simulink model "px4_6dof_quadrotor"  (R2021b)
settings: Solver=VariableStepAuto  StartTime=0.0  StopTime=10.0  RelTol=1e-3
undefined symbols (not defined in the file or in its folder): DiscIntNeverNeededParam, magnitude, rad, s
libraries: cstblocks x6, aerolibconvert2 x4, simulink x3, simulink_extras x3, sharedtransform x1, mspfiltlib x1, mspsensorlib x1
settings Model: Creator=user  LastModifiedBy=user

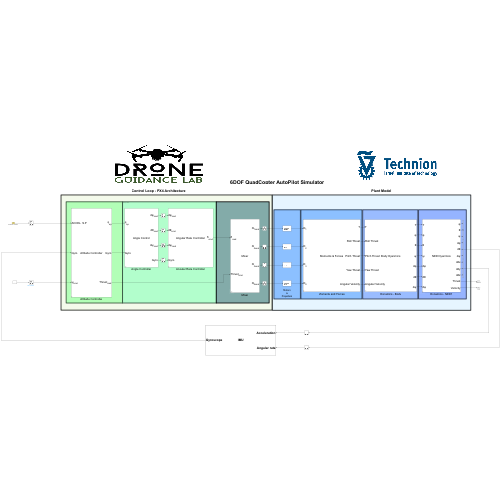
[thumbnail: Simulink's stored preview of the top-level diagram]
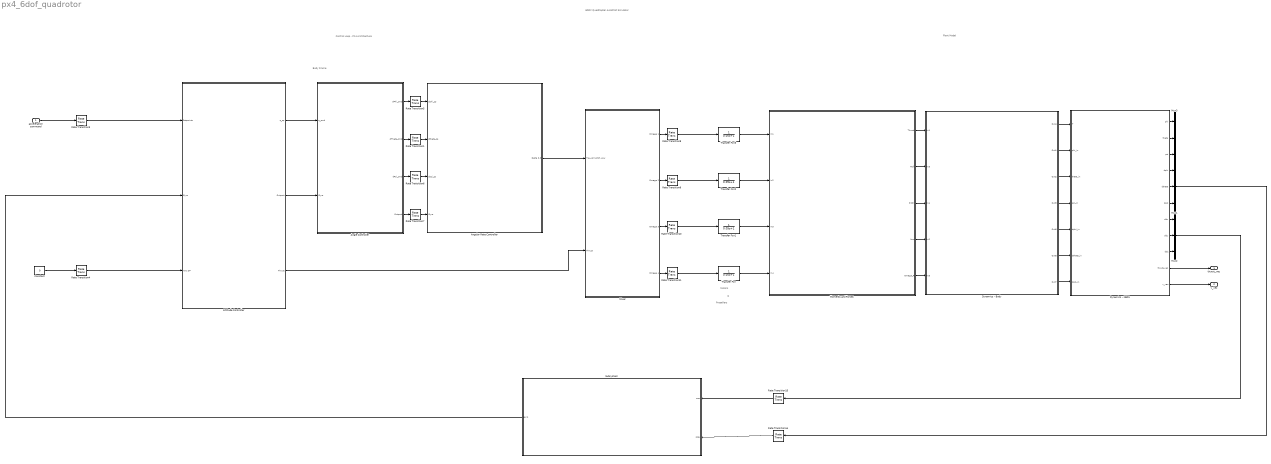
== system px4_6dof_quadrotor ==
  note: Control Loop - PX4 Architecture
  note: Body Frame
  note: Motors
  note: Plant Model
  note: 6DOF QuadCopter AutoPilot Simulator
  note: &
  note: Propellers
  acceleration command : Inport
  Angle Controller : Subsystem  mask{MC_ROLL_P=4, MC_PITCH_P=4, MC_YAW_P=4, MC_ROLLRATE_MAX=2, MC_PITCHRATE_MAX=2, MC_YAWRATE_MAX=2, MC_ACRO_R_MAX=2, MC_YAW_WEIGHT=0.1, m=0.9}
      mask prompts: MC_ROLL_P "MC_ROLL_P ="; MC_PITCH_P "MC_PITCH_P ="; MC_YAW_P "MC_YAW_P ="; MC_ROLLRATE_MAX "MC_ROLLRATE_MAX ="; MC_PITCHRATE_MAX "MC_PITCHRATE_MAX ="; MC_YAWRATE_MAX "MC_YAWRATE_MAX ="; MC_ACRO_R_MAX "MC_ACRO_R_MAX ="; MC_YAW_WEIGHT "MC_YAW_WEIGHT ="; m "m [kg] ="
      mask DialogControl DescTextVar Prompt: Attitude Controller - based on PX4 architecture
      mask Display:
      | disp('Angle Control')
      | 
      | port_label('input',1,'q_{sp}','texmode','on')
      | port_label('input',2,'Gyro')
      | 
      | port_label('output',1,'d\phi_{cmd}','texmode','on')
      | port_label('output',2,'d\theta_{cmd}','texmode','on')
      | port_label('output',3,'d\psi_{cmd}','texmode','on')
      | port_label('output',4,'Gyro','texmode','on')
  Angular Rate Controller : Subsystem  mask{MC_ROLLRATE_K=1, MC_ROLLRATE_P=0.044, MC_ROLLRATE_I=0.05, MC_ROLLRATE_D=0.0012, MC_RR_INT_LIM=101, MC_PITCHRATE_K=1, MC_PITCHRATE_P=0.044, MC_PITCHRATE_I=0.05, MC_PITCHRATE_D=0.0012, MC_PR_INT_LIM=100, MC_YAWRATE_K=1, MC_YAWRATE_P=0.044, MC_YAWRATE_I=0.05, MC_YAWRATE_D=0.0012, MC_YR_INT_LIM=100, IMU_DGYRO_CUTOFF=6000, IMU_GYRO_CUTOFF=0}
      mask prompts: MC_ROLLRATE_K "MC_ROLLRATE_K ="; MC_ROLLRATE_P "MC_ROLLRATE_P ="; MC_ROLLRATE_I "MC_ROLLRATE_I ="; MC_ROLLRATE_D "MC_ROLLRATE_D ="; MC_RR_INT_LIM "MC_RR_INT_LIM ="; MC_PITCHRATE_K "MC_PITCHRATE_K ="; MC_PITCHRATE_P "MC_PITCHRATE_P ="; MC_PITCHRATE_I "MC_PITCHRATE_I ="; MC_PITCHRATE_D "MC_PITCHRATE_D ="; MC_PR_INT_LIM "MC_PR_INT_LIM ="; MC_YAWRATE_K "MC_YAWRATE_K ="; MC_YAWRATE_P "MC_YAWRATE_P ="; MC_YAWRATE_I "MC_YAWRATE_I ="; MC_YAWRATE_D "MC_YAWRATE_D ="; MC_YR_INT_LIM "MC_YR_INT_LIM ="; IMU_DGYRO_CUTOFF "IMU_DGYRO_CUTOFF ="; IMU_GYRO_CUTOFF "IMU_GYRO_CUTOFF ="
      mask DialogControl DescTextVar Prompt: Angular rate controller, based on PX4 architecture
      mask DialogControl ROLL Prompt: Roll
      mask DialogControl PITCH Prompt: Pitch
      mask DialogControl YAW Prompt: Yaw
      mask Display:
      | disp('Angular Rate Controller')
      | 
      | port_label('input',1,'d\phi_{cmd}','texmode','on')
      | port_label('input',2,'d\theta_{cmd}','texmode','on')
      | port_label('input',3,'d\psi_{cmd}','texmode','on')
      | port_label('input',4,'Gyro','texmode','on')
      | 
      | port_label('output',1,'\delta_{cmd}','texmode','on')
  Attitude Controller : Subsystem  mask{MC_ROLL_P=1, MC_PITCH_P=5, MC_YAW_P=1, MC_ROLLRATE_MAX=2, MC_PITCHRATE_MAX=2, MC_YAWRATE_MAX=2, MC_ACRO_R_MAX=2, MC_YAW_WEIGHT=0.1, m=0.9}
      mask prompts: MC_ROLL_P "MC_ROLL_P ="; MC_PITCH_P "MC_PITCH_P ="; MC_YAW_P "MC_YAW_P ="; MC_ROLLRATE_MAX "MC_ROLLRATE_MAX ="; MC_PITCHRATE_MAX "MC_PITCHRATE_MAX ="; MC_YAWRATE_MAX "MC_YAWRATE_MAX ="; MC_ACRO_R_MAX "MC_ACRO_R_MAX ="; MC_YAW_WEIGHT "MC_YAW_WEIGHT ="; m "m [kg] ="
      mask DialogControl DescTextVar Prompt: Attitude Controller - based on PX4 architecture
      mask Display:
      | disp('Attitude Controller')
      | 
      | port_label('input',1,'ACCEL. S.P')
      | port_label('input',2,'Gyro')
      | port_label('input',3,'\psi_{cmd}','texmode','on')
      | 
      | port_label('output',1,'q_{sp}','texmode','on')
      | port_label('output',2,'Gyro','texmode','on')
      | port_label('output',3,'Thrust_{cmd}','texmode','on')
  Constant : Constant  Value=0
  Dynamics - Body : Subsystem  mask{Ixx=0.001, Iyy=0.001, Izz=0.0015, Jr=8e-7, d=0.165}
      mask prompts: Ixx "Ixx [kg*m^2] ="; Iyy "Iyy [kg*m^2] ="; Izz "Izz [kg*m^2]="; Jr "Jl [kg*m^2]="; d "d [m] ="
      mask DialogControl DescTextVar Prompt: This model represents the body-frame dyanmics. Enter the MOIs of the system
      mask Display:
      | disp('Body Dyanmics','texmode','on')
      | 
      | port_label('input',1,'T','texmode','on')
      | port_label('input',2,'Roll Thrust','texmode','on')
      | port_label('input',3,'Pitch Thrust','texmode','on')
      | port_label('input',4,'Yaw Thrust','texmode','on')
      | port_label('input',5,'Angular Velocity','texmode','on')
      | 
      | port_label('output',2,'\phi','texmode','on')
      | port_label('output',3,'\theta','texmode','on')
      | port_label('output',4,'\psi','texmode','on')
      | port_label('output',1,'T','texmode','on')
      | port_label('output',5,'d\phi','texmode','on')
      | port_label('output',6,'d\theta','texmode','on')
      | port_label('output',7,'d\psi','texmode','on')
  Dynamics - NED1 : Subsystem  mask{g=9.81, m=0.9, k=0.9}
      mask prompts: g "g [m/s^2] ="; m "m [kg] ="; k "k ="
      mask DialogControl DescTextVar Prompt: This block transform the body dyanmics to NED. Choose the mass, gravity, and Ax,Ay,Az - drag coeff.
      mask Display:
      | disp('NED Dyanmics','texmode','on')
      | 
      | port_label('input',2,'\phi','texmode','on')
      | port_label('input',3,'\theta','texmode','on')
      | port_label('input',4,'\psi','texmode','on')
      | port_label('input',1,'T','texmode','on')
      | port_label('input',5,'d\phi','texmode','on')
      | port_label('input',6,'d\theta','texmode','on')
      | port_label('input',7,'d\psi','texmode','on')
      | 
      | % port_label('output',1,'X','texmode','on')
      | % port_label('output',2,'Y','texmode','on')
      | % port_label('output',3,'Z','texmode','on')
      | 
      | % port_label('output',4,'dX','texmode','on')
      | % port_label('output',5,'dY','texmode','on')
      | % port_label('output',6,'dZ','texmode','on')
      | 
      | port_label('output',7,'ddx','texmode','on')
      | port_label('output',8,'ddy','texmode','on')
      | port_label('output',9,'ddz','texmode','on')
      | 
      | port_label('output',4,'d\phi','texmode','on')
      | port_label('output',5,'d\theta','texmode','on')
      | port_label('output',6,'d\psi','texmode','on')
      | 
      | port_label('output',1,'\phi','texmode','on')
      | port_label('output',2,'\theta','texmode','on')
      | port_label('output',3,'\psi','texmode','on')
      | 
      | port_label('output',10,'Thrust','texmode','on')
      | port_label('output',11,'Velocity','texmode','on')
  Mixer : Subsystem  mask{Ct=7e-6, Cq=1.6e-7, d=0.165}
      mask prompts: Ct "Ct ="; Cq "Cq ="; d "d [m] ="
      mask Display:
      | disp('Mixer')
      | 
      | port_label('input',1,'\delta_{cmd}','texmode','on')
      | port_label('input',2,'Thrust_{cmd}','texmode','on')
      | 
      | port_label('output',1,'\Omega_{1cmd}','texmode','on')
      | port_label('output',2,'\Omega_{2cmd}','texmode','on')
      | port_label('output',3,'\Omega_{3cmd}','texmode','on')
      | port_label('output',4,'\Omega_{4cmd}','texmode','on')
  Moments and Forces : Subsystem  mask{Ct=7e-6, Cq=1.6e-7, d=0.165, rpm_sat=15000}
      mask prompts: Ct "Ct ="; Cq "Cq ="; d "d [m] ="; rpm_sat "max motor speed [rpm]="
      mask DialogControl DescTextVar Prompt: This block represents the moment and force calculations. Supply the Ct - thrust constant and Cq is the drag consant. d is the quadrotor arm's length
      mask DialogControl Container3 Prompt: Constants:
      mask Display:
      | disp('Moments & Forces')
      | 
      | port_label('input',1,'\Omega_{1}','texmode','on')
      | port_label('input',2,'\Omega_{2}','texmode','on')
      | port_label('input',3,'\Omega_{3}','texmode','on')
      | port_label('input',4,'\Omega_{4}','texmode','on')
      | 
      | port_label('output',1,'T','texmode','on')
      | port_label('output',2,'Roll Thrust','texmode','on')
      | port_label('output',3,'Pitch Thrust','texmode','on')
      | port_label('output',4,'Yaw Thrust','texmode','on')
      | port_label('output',5,'Angular Velocity','texmode','on')
  Mux1 : Mux  Inputs=3
  Mux2 : Mux  Inputs=3
  Mux3 : Mux  Inputs=3
  Rate Transition{1,5..7} (4 alike) : RateTransition  OutPortSampleTime=1/1000
  Rate Transition{8..11} (4 alike) : RateTransition  OutPortSampleTime=1/10000
  Rate Transition14 : RateTransition  OutPortSampleTime=1/250
  Rate Transition15 : RateTransition  OutPortSampleTime=1/250
  Rate Transition3 : RateTransition  OutPortSampleTime=1/250
  Rate Transition4 : RateTransition  OutPortSampleTime=1/ 250
  Subsystem : Subsystem
      mask Display:
      | disp('IMU')
      | port_label('input',1,'Acceleration','texmode','on')
      | port_label('input',2,'Angular rate','texmode','on')
      | port_label('output',1,'Gyroscope','texmode','on')
  Transfer Fcn{,1..3} (4 alike) : TransferFcn  Denominator=[0.05 1]
  thurst_vec : Outport
  v_vec : Outport  Port=2
  wires:
  Moments and Forces/1(Thrust) -> Dynamics - Body/1(In1)
  Transfer Fcn/1 -> Moments and Forces/4(In4)
  Rate Transition15/1 -> Subsystem/1(acc)
  Mux1/1 -> Rate Transition14/1
  Subsystem/1(gyro) -> Attitude Controller/2(Gyro)
  Dynamics - NED1/1(phi) -> Mux3/1
  Dynamics - NED1/6(dpsi) -> Mux1/3
  Attitude Controller/2(Outport) -> Angle Controller/2(Gyro)
  Rate Transition9/1 -> Transfer Fcn2/1
  Dynamics - NED1/2(theta) -> Mux3/2
  Mixer/1(Omega 1) -> Rate Transition8/1
  Rate Transition10/1 -> Transfer Fcn1/1
  Dynamics - NED1/4(dphi) -> Mux1/1
  Dynamics - NED1/9(ddz) -> Mux2/3
  Rate Transition14/1 -> Subsystem/2(rate)
  Rate Transition5/1 -> Angular Rate Controller/1(dphi_sp)
  Angle Controller/2(dTheta_cmd) -> Rate Transition1/1
  Rate Transition6/1 -> Angular Rate Controller/3(dpsi_sp)
  Dynamics - NED1/5(dtheta) -> Mux1/2
  Angle Controller/3(dPsi_cmd) -> Rate Transition6/1
  Rate Transition3/1 -> Attitude Controller/1(Setpoints)
  Dynamics - NED1/3(psi) -> Mux3/3
  Transfer Fcn1/1 -> Moments and Forces/3(In3)
  Rate Transition11/1 -> Transfer Fcn/1
  Transfer Fcn3/1 -> Moments and Forces/1(In1)
  Transfer Fcn2/1 -> Moments and Forces/2(In2)
  Dynamics - Body/4(Out3) -> Dynamics - NED1/4(psi_in)
  Moments and Forces/5(Omega_R) -> Dynamics - Body/5(In5)
  Rate Transition1/1 -> Angular Rate Controller/2(dtheta_sp)
  Mixer/3(Omega 3) -> Rate Transition10/1
  Rate Transition4/1 -> Attitude Controller/3(Yaw.SP)
  acceleration command/1 -> Rate Transition3/1
  Dynamics - Body/1(Out4) -> Dynamics - NED1/1(T)
  Dynamics - NED1/8(ddy) -> Mux2/2
  Attitude Controller/1(q_sp) -> Angle Controller/1(q_cmd)
  Constant/1 -> Rate Transition4/1
  Dynamics - Body/7(Out7) -> Dynamics - NED1/7(dpsi_in)
  Angular Rate Controller/1(Delta S.P) -> Mixer/1(Tau_roll,pitch,yaw)
  Moments and Forces/4(Yaw) -> Dynamics - Body/4(In2)
  Angle Controller/4(Outport) -> Rate Transition7/1
  Dynamics - Body/6(Out6) -> Dynamics - NED1/6(dtheta_in)
  Rate Transition8/1 -> Transfer Fcn3/1
  Dynamics - Body/5(Out5) -> Dynamics - NED1/5(dphi_in)
  Mixer/4(Omega 4) -> Rate Transition11/1
  Dynamics - NED1/11(v_vec) -> v_vec/1
  Dynamics - NED1/10(thrust_vec) -> thurst_vec/1
  Attitude Controller/3(Thrust) -> Mixer/2(Thrust)
  Dynamics - NED1/7(ddx) -> Mux2/1
  Moments and Forces/3(Pitch) -> Dynamics - Body/3(In4)
  Dynamics - Body/3(Out2) -> Dynamics - NED1/3(theta_in)
  Mixer/2(Omega 2) -> Rate Transition9/1
  Moments and Forces/2(Roll) -> Dynamics - Body/2(In3)
  Mux2/1 -> Rate Transition15/1
  Angle Controller/1(dPhi_cmd) -> Rate Transition5/1
  Dynamics - Body/2(Out1) -> Dynamics - NED1/2(phi_in)
  Rate Transition7/1 -> Angular Rate Controller/4(Gyro)

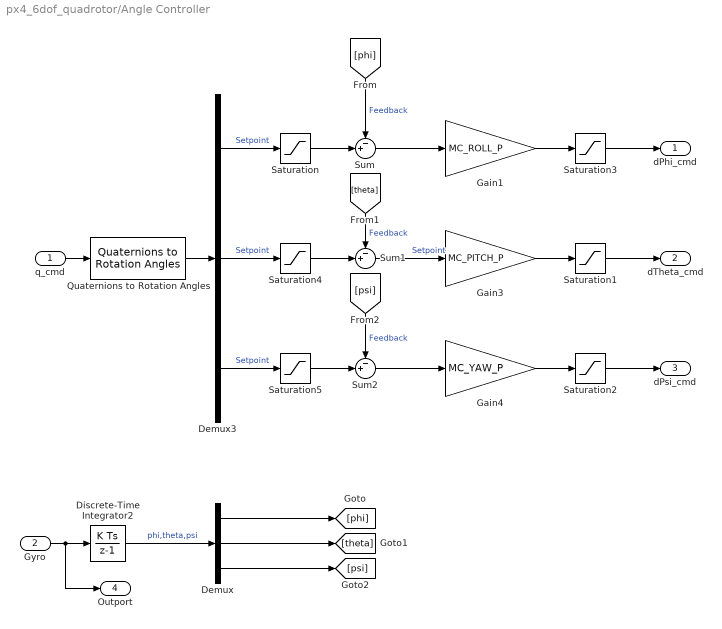
== system px4_6dof_quadrotor/Angle Controller ==
  q_cmd : Inport
  Gyro : Inport  Port=2
  Demux : Demux  Outputs=3
  Demux3 : Demux  Outputs=3
  Discrete-Time Integrator2 : DiscreteIntegrator  InitialCondition=[0.001;0.001;0.001]  SampleTime=-1  ICPrevOutput=DiscIntNeverNeededParam  ICPrevScaledInput=DiscIntNeverNeededParam
  Gain1 : Gain  Gain=MC_ROLL_P
  Gain3 : Gain  Gain=MC_PITCH_P
  Gain4 : Gain  Gain=MC_YAW_P
  Quaternions to Rotation Angles : sharedtransform/Quaternions to Rotation Angles  rotationOrder=XYZ  aMode=aMode
      settings: SourceProductBaseCode=AE,PW,DR,MT,UV,VE
  Saturation : Saturate  UpperLimit=1.5  LowerLimit=-1.5
  Saturation1 : Saturate  UpperLimit=MC_PITCHRATE_MAX  LowerLimit=-MC_PITCHRATE_MAX
  Saturation2 : Saturate  UpperLimit=MC_YAWRATE_MAX  LowerLimit=-MC_YAWRATE_MAX
  Saturation3 : Saturate  UpperLimit=MC_ROLLRATE_MAX  LowerLimit=-MC_ROLLRATE_MAX
  Saturation4 : Saturate  UpperLimit=1.5  LowerLimit=-1.5
  Saturation5 : Saturate  UpperLimit=1.5  LowerLimit=-1.5
  Sum : Sum  Inputs=-+|
  Sum1 : Sum  Inputs=-+|
  Sum2 : Sum  Inputs=-+|
  dPhi_cmd : Outport
  dTheta_cmd : Outport  Port=2
  dPsi_cmd : Outport  Port=3
  Outport : Outport  Port=4
  wires:
  Discrete-Time Integrator2/1 -> Demux/1  "phi,theta,psi"
  Gyro/1 -> Outport/1, Discrete-Time Integrator2/1
  Demux/2 -> [theta]
  Demux/1 -> [phi]
  Demux/3 -> [psi]
  Demux3/1 -> Saturation/1  "Setpoint"
  Demux3/2 -> Saturation4/1  "Setpoint"
  Demux3/3 -> Saturation5/1  "Setpoint"
  Saturation3/1 -> dPhi_cmd/1
  Gain1/1 -> Saturation3/1
  Gain3/1 -> Saturation1/1
  Gain4/1 -> Saturation2/1
  Saturation1/1 -> dTheta_cmd/1
  Saturation2/1 -> dPsi_cmd/1
  [phi] -> Sum/1  "Feedback"
  Sum/1 -> Gain1/1
  [theta] -> Sum1/1  "Feedback"
  Sum2/1 -> Gain4/1
  [psi] -> Sum2/1  "Feedback"
  Sum1/1 -> Gain3/1  "Setpoint"
  q_cmd/1 -> Quaternions to Rotation Angles/1
  Quaternions to Rotation Angles/1 -> Demux3/1
  Saturation/1 -> Sum/2
  Saturation4/1 -> Sum1/2
  Saturation5/1 -> Sum2/2

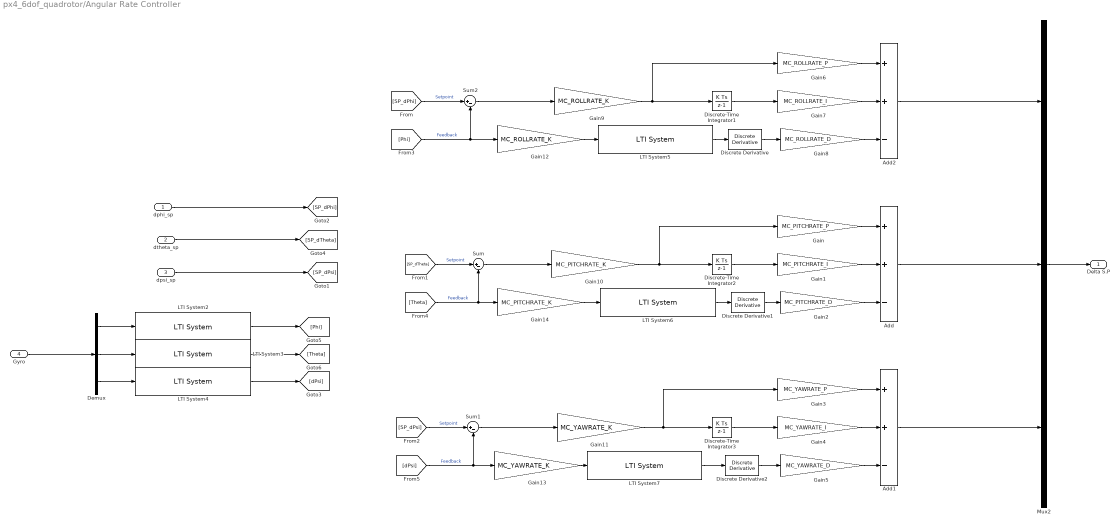
== system px4_6dof_quadrotor/Angular Rate Controller ==
  dphi_sp : Inport
  dtheta_sp : Inport  Port=2
  dpsi_sp : Inport  Port=3
  Gyro : Inport  Port=4
  Add : Sum  Inputs=++-
  Add1 : Sum  Inputs=++-
  Add2 : Sum  Inputs=++-
  Demux : Demux  Outputs=3
  Discrete Derivative : simulink/Discrete/Discrete Derivative  gainval=1.0  ICPrevScaledInput=0.0  OutMin=[]  OutMax=[]  OutDataType=fixdt(1, 16)  OutScaling=2^-10  DoSatur=off
  Discrete Derivative1 : simulink/Discrete/Discrete Derivative  gainval=1.0  ICPrevScaledInput=0.0  OutMin=[]  OutMax=[]  OutDataType=fixdt(1, 16)  OutScaling=2^-10  DoSatur=off
  Discrete Derivative2 : simulink/Discrete/Discrete Derivative  gainval=1.0  ICPrevScaledInput=0.0  OutMin=[]  OutMax=[]  OutDataType=fixdt(1, 16)  OutScaling=2^-10  DoSatur=off
  Discrete-Time Integrator1 : DiscreteIntegrator  SampleTime=1/1000  LimitOutput=on  UpperSaturationLimit=MC_RR_INT_LIM  LowerSaturationLimit=-MC_RR_INT_LIM  ICPrevOutput=DiscIntNeverNeededParam  ICPrevScaledInput=DiscIntNeverNeededParam
  Discrete-Time Integrator2 : DiscreteIntegrator  SampleTime=1/1000  LimitOutput=on  UpperSaturationLimit=MC_PR_INT_LIM  LowerSaturationLimit=-MC_PR_INT_LIM  ICPrevOutput=DiscIntNeverNeededParam  ICPrevScaledInput=DiscIntNeverNeededParam
  Discrete-Time Integrator3 : DiscreteIntegrator  SampleTime=1/1000  LimitOutput=on  UpperSaturationLimit=MC_YR_INT_LIM  LowerSaturationLimit=-MC_YR_INT_LIM  ICPrevOutput=DiscIntNeverNeededParam  ICPrevScaledInput=DiscIntNeverNeededParam
  Gain : Gain  Gain=MC_PITCHRATE_P
  Gain1 : Gain  Gain=MC_PITCHRATE_I
  Gain10 : Gain  Gain=MC_PITCHRATE_K
  Gain11 : Gain  Gain=MC_YAWRATE_K
  Gain12 : Gain  Gain=MC_ROLLRATE_K
  Gain13 : Gain  Gain=MC_YAWRATE_K
  Gain14 : Gain  Gain=MC_PITCHRATE_K
  Gain2 : Gain  Gain=MC_PITCHRATE_D
  Gain3 : Gain  Gain=MC_YAWRATE_P
  Gain4 : Gain  Gain=MC_YAWRATE_I
  Gain5 : Gain  Gain=MC_YAWRATE_D
  Gain6 : Gain  Gain=MC_ROLLRATE_P
  Gain7 : Gain  Gain=MC_ROLLRATE_I
  Gain8 : Gain  Gain=MC_ROLLRATE_D
  Gain9 : Gain  Gain=MC_ROLLRATE_K
  LTI System2 : cstblocks/LTI System  sys=c2d(tf(1,[IMU_GYRO_CUTOFF 1]),1/1000)  IC=[]
  LTI System3 : cstblocks/LTI System  sys=c2d(tf(1,[IMU_GYRO_CUTOFF 1]),1/1000)  IC=[]
  LTI System4 : cstblocks/LTI System  sys=c2d(tf(1,[IMU_GYRO_CUTOFF 1]),1/1000)  IC=[]
  LTI System5 : cstblocks/LTI System  sys=c2d(tf(1,[IMU_DGYRO_CUTOFF 1]),1/1000)  IC=[]
  LTI System6 : cstblocks/LTI System  sys=c2d(tf(1,[IMU_DGYRO_CUTOFF 1]),1/1000)  IC=[]
  LTI System7 : cstblocks/LTI System  sys=c2d(tf(1,[IMU_DGYRO_CUTOFF 1]),1/1000)  IC=[]
  Mux2 : Mux  Inputs=3
  Sum : Sum  Inputs=|+-
  Sum1 : Sum  Inputs=|+-
  Sum2 : Sum  Inputs=|+-
  Delta S.P : Outport
  wires:
  dtheta_sp/1 -> [SP_dTheta]
  LTI System6/1 -> Discrete Derivative1/1
  Sum/1 -> Gain10/1
  Discrete-Time Integrator2/1 -> Gain1/1
  Gain2/1 -> Add/3
  Gain1/1 -> Add/2
  Gain/1 -> Add/1
  Gain3/1 -> Add1/1
  Gain4/1 -> Add1/2
  Gain5/1 -> Add1/3
  Discrete-Time Integrator3/1 -> Gain4/1
  Sum1/1 -> Gain11/1
  LTI System7/1 -> Discrete Derivative2/1
  [dPsi] -> Gain13/1, Sum1/2  "Feedback"
  [SP_dPsi] -> Sum1/1  "Setpoint"
  Add/1 -> Mux2/2
  Mux2/1 -> Delta S.P/1
  Gain6/1 -> Add2/1
  Gain7/1 -> Add2/2
  Gain8/1 -> Add2/3
  Discrete-Time Integrator1/1 -> Gain7/1
  Sum2/1 -> Gain9/1
  LTI System5/1 -> Discrete Derivative/1
  [SP_dPhi] -> Sum2/1  "Setpoint"
  [SP_dTheta] -> Sum/1  "Setpoint"
  [Phi] -> Gain12/1, Sum2/2  "Feedback"
  [Theta] -> Gain14/1, Sum/2  "Feedback"
  Add1/1 -> Mux2/3
  Discrete Derivative/1 -> Gain8/1
  Discrete Derivative1/1 -> Gain2/1
  Discrete Derivative2/1 -> Gain5/1
  Gain9/1 -> Discrete-Time Integrator1/1, Gain6/1
  Gain10/1 -> Discrete-Time Integrator2/1, Gain/1
  Gain11/1 -> Discrete-Time Integrator3/1, Gain3/1
  Gain12/1 -> LTI System5/1
  Gain13/1 -> LTI System7/1
  Gain14/1 -> LTI System6/1
  Gyro/1 -> Demux/1
  Demux/1 -> LTI System2/1
  Demux/2 -> LTI System3/1
  Demux/3 -> LTI System4/1
  LTI System2/1 -> [Phi]
  LTI System3/1 -> [Theta]
  LTI System4/1 -> [dPsi]
  dpsi_sp/1 -> [SP_dPsi]
  dphi_sp/1 -> [SP_dPhi]
  Add2/1 -> Mux2/1

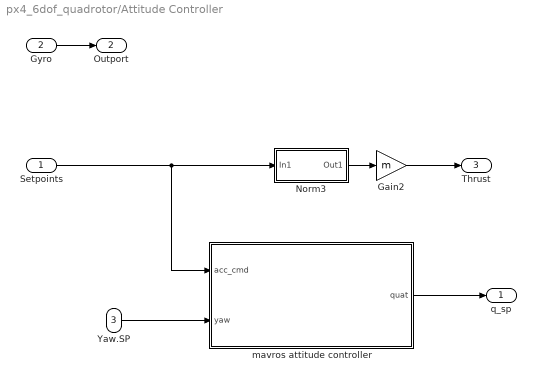
== system px4_6dof_quadrotor/Attitude Controller ==
  Setpoints : Inport
  Gyro : Inport  Port=2
  Yaw.SP : Inport  Port=3
  Gain2 : Gain  Gain=m
  Norm3 : Subsystem
      mask Display: disp('Norm')
  mavros attitude controller : Subsystem
      mask Display:
      | disp('Mavros Geometric controller')
      | port_label('input',1,'acc_{cmd}','texmode','on')
      | port_label('input',2,'\psi_{cmd}','texmode','on')
      | 
      | 
      | port_label('output',1,'quat','texmode','on')
  q_sp : Outport
  Outport : Outport  Port=2
  Thrust : Outport  Port=3
  wires:
  Norm3/1(Out1) -> Gain2/1
  Gain2/1 -> Thrust/1
  Yaw.SP/1 -> mavros attitude controller/2(yaw)
  mavros attitude controller/1(quat) -> q_sp/1
  Setpoints/1 -> mavros attitude controller/1(acc_cmd), Norm3/1(In1)
  Gyro/1 -> Outport/1

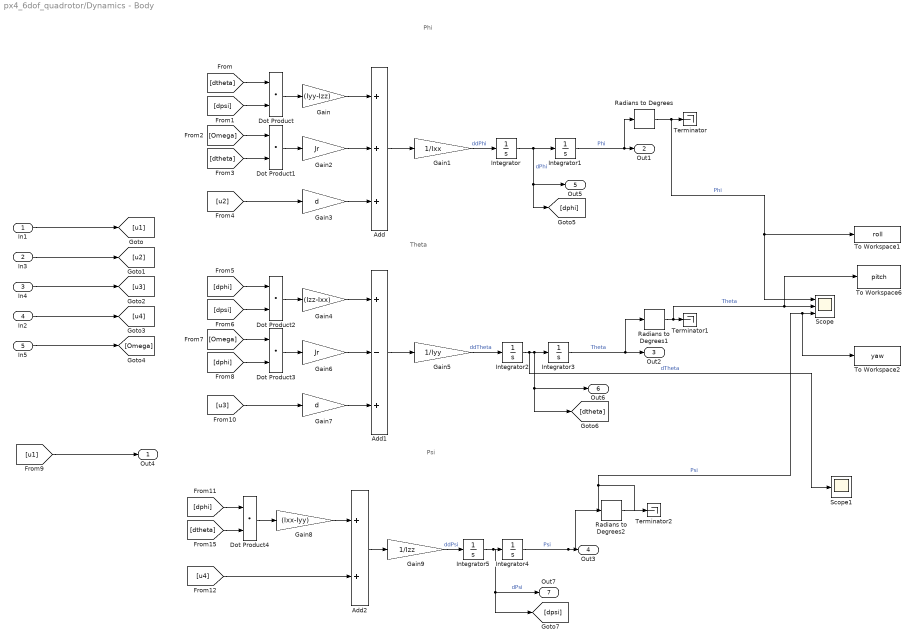
== system px4_6dof_quadrotor/Dynamics - Body ==
  note: Phi
  note: Theta
  note: Psi
  In1 : Inport
  In3 : Inport  Port=2
  In4 : Inport  Port=3
  In2 : Inport  Port=4
  In5 : Inport  Port=5
  Add : Sum  Inputs=3
  Add1 : Sum  Inputs=+-+
  Add2 : Sum  Inputs=2
  Dot Product{,1..4} (5 alike) : DotProduct  InputSameDT=on  OutDataTypeStr=Inherit: Inherit via internal rule
  Gain : Gain  Gain=(Iyy-Izz)
  Gain1 : Gain  Gain=1/Ixx
  Gain2 : Gain  Gain=Jr
  Gain3 : Gain  Gain=d
  Gain4 : Gain  Gain=(Izz-Ixx)
  Gain5 : Gain  Gain=1/Iyy
  Gain6 : Gain  Gain=Jr
  Gain7 : Gain  Gain=d
  Gain8 : Gain  Gain=(Ixx-Iyy)
  Gain9 : Gain  Gain=1/Izz
  Integrator{,1..5} (6 alike) : Integrator
  Radians to Degrees : simulink_extras/Transformations/Radians to Degrees
  Radians to Degrees1 : simulink_extras/Transformations/Radians to Degrees
  Radians to Degrees2 : simulink_extras/Transformations/Radians to Degrees
  Scope : Scope  NumInputPorts=3
  Scope1 : Scope
  Terminator : Terminator
  Terminator1 : Terminator
  Terminator2 : Terminator
  To Workspace1 : ToWorkspace  VariableName=roll  SampleTime=-1
  To Workspace2 : ToWorkspace  VariableName=yaw  SampleTime=-1
  To Workspace6 : ToWorkspace  VariableName=pitch  SampleTime=-1
  Out4 : Outport
  Out1 : Outport  Port=2
  Out2 : Outport  Port=3
  Out3 : Outport  Port=4
  Out5 : Outport  Port=5
  Out6 : Outport  Port=6
  Out7 : Outport  Port=7
  wires:
  In1/1 -> [u1]
  In3/1 -> [u2]
  In4/1 -> [u3]
  In2/1 -> [u4]
  In5/1 -> [Omega]
  Integrator/1 -> [dphi], Out5/1, Integrator1/1  "dPhi"
  Integrator2/1 -> Scope1/1, Integrator3/1, [dtheta], Out6/1  "dTheta"
  Integrator5/1 -> [dpsi], Out7/1, Integrator4/1  "dPsi"
  Integrator1/1 -> Out1/1, Radians to Degrees/1  "Phi"
  Integrator3/1 -> Radians to Degrees1/1, Out2/1  "Theta"
  Integrator4/1 -> Radians to Degrees2/1, Out3/1  "Psi"
  [dpsi] -> Dot Product/2
  [dtheta] -> Dot Product/1
  Dot Product/1 -> Gain/1
  Gain/1 -> Add/1
  Gain1/1 -> Integrator/1  "ddPhi"
  Add/1 -> Gain1/1
  [Omega] -> Dot Product1/1
  Dot Product1/1 -> Gain2/1
  [dtheta] -> Dot Product1/2
  Gain2/1 -> Add/2
  [u2] -> Gain3/1
  Gain7/1 -> Add1/3
  [u3] -> Gain7/1
  Gain6/1 -> Add1/2
  [dphi] -> Dot Product3/2
  Dot Product3/1 -> Gain6/1
  [Omega] -> Dot Product3/1
  Add1/1 -> Gain5/1
  Gain4/1 -> Add1/1
  Dot Product2/1 -> Gain4/1
  [dphi] -> Dot Product2/1
  [dpsi] -> Dot Product2/2
  Gain5/1 -> Integrator2/1  "ddTheta"
  [dtheta] -> Dot Product4/2
  Dot Product4/1 -> Gain8/1
  Gain8/1 -> Add2/1
  Add2/1 -> Gain9/1
  Gain9/1 -> Integrator5/1  "ddPsi"
  [dphi] -> Dot Product4/1
  [u4] -> Add2/2
  [u1] -> Out4/1
  Gain3/1 -> Add/3
  Radians to Degrees/1 -> Scope/1, To Workspace1/1, Terminator/1  "Phi"
  Radians to Degrees1/1 -> To Workspace6/1, Scope/2, Terminator1/1  "Theta"
  Radians to Degrees2/1 -> Terminator2/1, To Workspace2/1, Scope/3  "Psi"

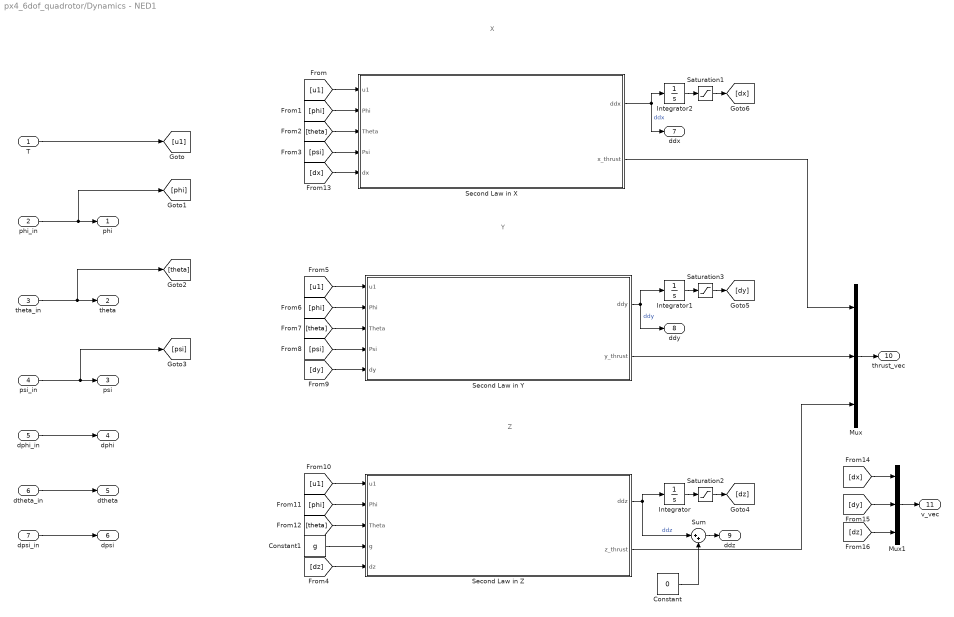
== system px4_6dof_quadrotor/Dynamics - NED1 ==
  note: X
  note: Y
  note: Z
  T : Inport
  phi_in : Inport  Port=2
  theta_in : Inport  Port=3
  psi_in : Inport  Port=4
  dphi_in : Inport  Port=5
  dtheta_in : Inport  Port=6
  dpsi_in : Inport  Port=7
  Constant : Constant  Value=0
  Constant1 : Constant  Value=g  SampleTime=-1
  Integrator : Integrator
  Integrator1 : Integrator
  Integrator2 : Integrator
  Mux : Mux  Inputs=3
  Mux1 : Mux  Inputs=3
  Saturation1 : Saturate  UpperLimit=50  LowerLimit=-50
  Saturation2 : Saturate  UpperLimit=50  LowerLimit=-50
  Saturation3 : Saturate  UpperLimit=50  LowerLimit=-50
  Second Law in X : Subsystem
  Second Law in Y : Subsystem
  Second Law in Z : Subsystem
  Sum : Sum  Inputs=|++
  phi : Outport
  theta : Outport  Port=2
  psi : Outport  Port=3
  dphi : Outport  Port=4
  dtheta : Outport  Port=5
  dpsi : Outport  Port=6
  ddx : Outport  Port=7
  ddy : Outport  Port=8
  ddz : Outport  Port=9
  thrust_vec : Outport  Port=10
  v_vec : Outport  Port=11
  wires:
  dpsi_in/1 -> dpsi/1
  dtheta_in/1 -> dtheta/1
  dphi_in/1 -> dphi/1
  psi_in/1 -> [psi], psi/1
  theta_in/1 -> [theta], theta/1
  phi_in/1 -> [phi], phi/1
  T/1 -> [u1]
  Second Law in X/1(ddx) -> ddx/1, Integrator2/1  "ddx"
  [u1] -> Second Law in X/1(u1)
  [phi] -> Second Law in X/2(Phi)
  [theta] -> Second Law in X/3(Theta)
  [psi] -> Second Law in X/4(Psi)
  [psi] -> Second Law in Y/4(Psi)
  [theta] -> Second Law in Y/3(Theta)
  [phi] -> Second Law in Y/2(Phi)
  [u1] -> Second Law in Y/1(u1)
  Second Law in Y/1(ddy) -> ddy/1, Integrator1/1  "ddy"
  Second Law in Z/1(ddz) -> Sum/1, Integrator/1  "ddz"
  [u1] -> Second Law in Z/1(u1)
  [phi] -> Second Law in Z/2(Phi)
  [theta] -> Second Law in Z/3(Theta)
  Constant1/1 -> Second Law in Z/4(g)
  [dz] -> Second Law in Z/5(dz)
  [dy] -> Second Law in Y/5(dy)
  [dx] -> Second Law in X/5(dx)
  Integrator/1 -> Saturation2/1
  Integrator1/1 -> Saturation3/1
  Integrator2/1 -> Saturation1/1
  Saturation1/1 -> [dx]
  Saturation3/1 -> [dy]
  Saturation2/1 -> [dz]
  Second Law in X/2(x_thrust) -> Mux/1
  Second Law in Y/2(y_thrust) -> Mux/2
  Second Law in Z/2(z_thrust) -> Mux/3
  Mux/1 -> thrust_vec/1
  Mux1/1 -> v_vec/1
  [dx] -> Mux1/1
  [dy] -> Mux1/2
  [dz] -> Mux1/3
  Sum/1 -> ddz/1
  Constant/1 -> Sum/2

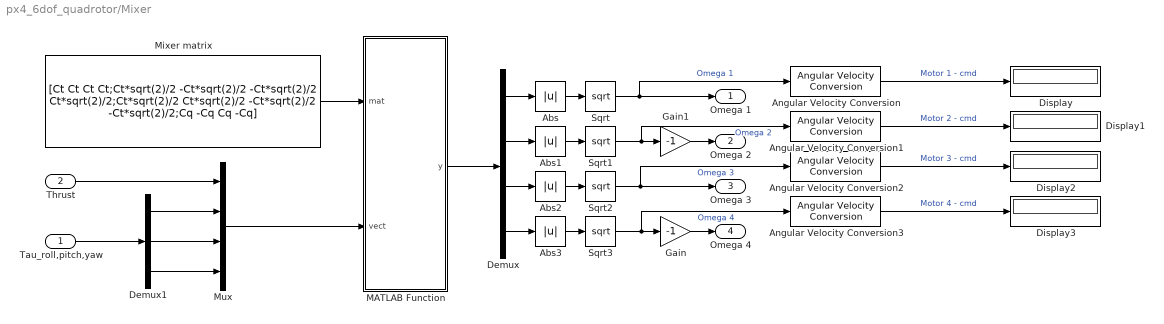
== system px4_6dof_quadrotor/Mixer ==
  Tau_roll,pitch,yaw : Inport
  Thrust : Inport  Port=2
  Abs{,1..3} (4 alike) : Abs
  Angular Velocity Conversion{,1..3} (4 alike) : aerolibconvert2/Angular Velocity Conversion  IU=rad/s  OU=rpm
  Demux : Demux
  Demux1 : Demux  Outputs=3
  Display{,1..3} (4 alike) : Display
  Gain : Gain  Gain=-1
  Gain1 : Gain  Gain=-1
  MATLAB Function : MATLAB Function  TreatAsAtomicUnit=on
  Mixer matrix : Constant  StartFcn=|  Value=[Ct Ct Ct Ct;Ct*sqrt(2)/2 -Ct*sqrt(2)/2 -Ct*sqrt(2)/2 Ct*sqrt(2)/2;Ct*sqrt(2)/2 Ct*sqrt(2)/2 -Ct*sqrt(2)/2 -Ct*sqrt(2)/2;Cq -Cq Cq -Cq]  OutDataTypeStr=Inherit: Inherit via back propagation  SampleTime=1/1000
      | %p = Simulink.Mask.get('ControlsModels/Moments and Forces');
      | 
      | Ct = 0.025
      | Cq = 2e-6;
      | 
      | %Ct = p.getParameter('Ct');
      | %Cq =p.getParameter('Cq');
      | 
      | %Ct = str2double(Ct.Value);
      | %Cq = str2double(Cq.Value);
  Mux : Mux
  Sqrt{,1..3} (4 alike) : Sqrt  SaturateOnIntegerOverflow=on
  Omega 1 : Outport
  Omega 2 : Outport  Port=2
  Omega 3 : Outport  Port=3
  Omega 4 : Outport  Port=4
  wires:
  Thrust/1 -> Mux/1
  Demux/1 -> Abs/1
  Demux/2 -> Abs1/1
  Demux/3 -> Abs2/1
  Demux/4 -> Abs3/1
  MATLAB Function/1(y) -> Demux/1
  Mux/1 -> MATLAB Function/2(vect)
  Mixer matrix/1 -> MATLAB Function/1(mat)
  Sqrt/1 -> Angular Velocity Conversion/1, Omega 1/1  "Omega 1"
  Sqrt1/1 -> Angular Velocity Conversion1/1, Gain1/1  "Omega 2"
  Sqrt2/1 -> Angular Velocity Conversion2/1, Omega 3/1  "Omega 3"
  Sqrt3/1 -> Angular Velocity Conversion3/1, Gain/1  "Omega 4"
  Tau_roll,pitch,yaw/1 -> Demux1/1
  Demux1/3 -> Mux/4
  Demux1/1 -> Mux/2
  Demux1/2 -> Mux/3
  Angular Velocity Conversion/1 -> Display/1  "Motor 1 - cmd"
  Angular Velocity Conversion1/1 -> Display1/1  "Motor 2 - cmd"
  Angular Velocity Conversion2/1 -> Display2/1  "Motor 3 - cmd"
  Angular Velocity Conversion3/1 -> Display3/1  "Motor 4 - cmd"
  Abs/1 -> Sqrt/1
  Abs1/1 -> Sqrt1/1
  Abs2/1 -> Sqrt2/1
  Abs3/1 -> Sqrt3/1
  Gain/1 -> Omega 4/1
  Gain1/1 -> Omega 2/1

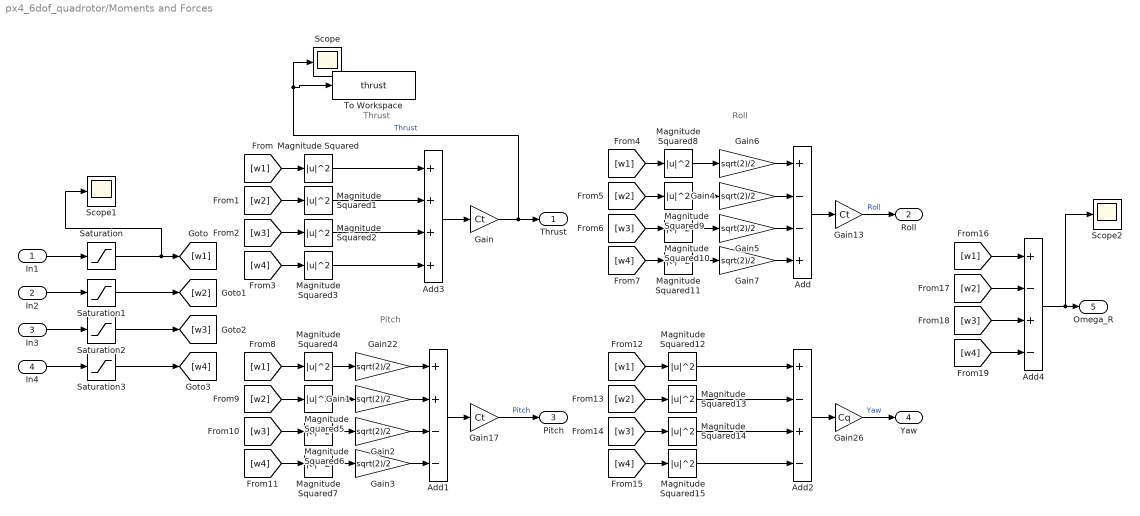
== system px4_6dof_quadrotor/Moments and Forces ==
  note: Thrust
  note: Roll
  note: Pitch
  In1 : Inport
  In2 : Inport  Port=2
  In3 : Inport  Port=3
  In4 : Inport  Port=4
  Add : Sum  Inputs=+--+
  Add1 : Sum  Inputs=++--
  Add2 : Sum  Inputs=+-+-
  Add3 : Sum  Inputs=4
  Add4 : Sum  Inputs=+-+-
  Gain : Gain  Gain=Ct
  Gain{1..7,22} (8 alike) : Gain  Gain=sqrt(2)/2
  Gain13 : Gain  Gain=Ct
  Gain17 : Gain  Gain=Ct
  Gain26 : Gain  Gain=Cq
  Magnitude Squared{,1..15} (16 alike) : Math  Operator=magnitude^2  SaturateOnIntegerOverflow=on
  Saturation{,1..3} (4 alike) : Saturate  UpperLimit=rpm_sat*(pi/30)  LowerLimit=-rpm_sat*(pi/30)
  Scope : Scope
  Scope1 : Scope
  Scope2 : Scope
  To Workspace : ToWorkspace  VariableName=thrust  SaveFormat=Timeseries  SampleTime=-1
  Thrust : Outport
  Roll : Outport  Port=2
  Pitch : Outport  Port=3
  Yaw : Outport  Port=4
  Omega_R : Outport  Port=5
  wires:
  In1/1 -> Saturation/1
  In2/1 -> Saturation1/1
  In3/1 -> Saturation2/1
  In4/1 -> Saturation3/1
  [w1] -> Magnitude Squared/1
  [w2] -> Magnitude Squared1/1
  [w3] -> Magnitude Squared2/1
  [w4] -> Magnitude Squared3/1
  Gain/1 -> To Workspace/1, Scope/1, Thrust/1  "Thrust"
  [w1] -> Magnitude Squared8/1
  [w2] -> Magnitude Squared9/1
  [w3] -> Magnitude Squared10/1
  [w4] -> Magnitude Squared11/1
  Add/1 -> Gain13/1
  Gain13/1 -> Roll/1  "Roll"
  Gain17/1 -> Pitch/1  "Pitch"
  [w4] -> Magnitude Squared7/1
  [w3] -> Magnitude Squared6/1
  [w2] -> Magnitude Squared5/1
  [w1] -> Magnitude Squared4/1
  Gain26/1 -> Yaw/1  "Yaw"
  Add2/1 -> Gain26/1
  Add3/1 -> Gain/1
  Gain1/1 -> Add1/2
  Gain3/1 -> Add1/4
  Gain2/1 -> Add1/3
  Gain22/1 -> Add1/1
  Add1/1 -> Gain17/1
  Gain5/1 -> Add/3
  Gain4/1 -> Add/2
  Gain6/1 -> Add/1
  Gain7/1 -> Add/4
  [w1] -> Magnitude Squared12/1
  [w3] -> Magnitude Squared14/1
  [w4] -> Magnitude Squared15/1
  [w2] -> Magnitude Squared13/1
  Magnitude Squared/1 -> Add3/1
  Magnitude Squared1/1 -> Add3/2
  Magnitude Squared2/1 -> Add3/3
  Magnitude Squared3/1 -> Add3/4
  Magnitude Squared4/1 -> Gain22/1
  Magnitude Squared7/1 -> Gain3/1
  Magnitude Squared6/1 -> Gain2/1
  Magnitude Squared5/1 -> Gain1/1
  Magnitude Squared11/1 -> Gain7/1
  Magnitude Squared10/1 -> Gain5/1
  Magnitude Squared8/1 -> Gain6/1
  Magnitude Squared9/1 -> Gain4/1
  Magnitude Squared12/1 -> Add2/1
  Magnitude Squared13/1 -> Add2/2
  Magnitude Squared14/1 -> Add2/3
  Magnitude Squared15/1 -> Add2/4
  [w2] -> Add4/2
  [w1] -> Add4/1
  [w3] -> Add4/3
  [w4] -> Add4/4
  Add4/1 -> Scope2/1, Omega_R/1
  Saturation/1 -> Scope1/1, [w1]
  Saturation1/1 -> [w2]
  Saturation3/1 -> [w4]
  Saturation2/1 -> [w3]

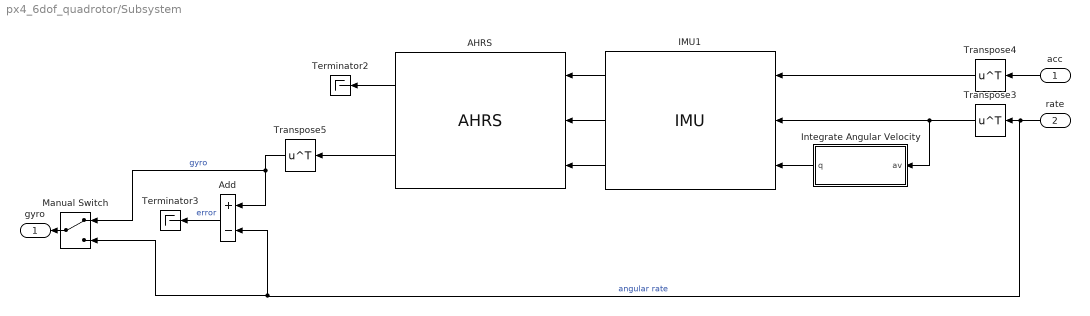
== system px4_6dof_quadrotor/Subsystem ==
  acc : Inport
  rate : Inport  Port=2
  AHRS : mspfiltlib/AHRS  DispRefFrame=NED  DecimationFactor=1  InitialProcessNoise=ahrsfilter.defaultProcessNoise  OrientationFormat=quaternion  SimulateUsing=Code generation  AccelerometerNoise=0.0001924722  GyroscopeNoise=9.1385e-5  MagnetometerNoise=0.1  GyroscopeDriftNoise=3.0462e-13  LinearAccelerationNoise=0.0096236100000000012  MagneticDisturbanceNoise=0.5  LinearAccelerationDecayFactor=0.5  MagneticDisturbanceDecayFactor=0.5  ExpectedMagneticFieldStrength=50
      settings: SourceProductName=Sensor Fusion and Tracking Toolbox
  Add : Sum  Inputs=+-
  IMU1 : mspsensorlib/IMU  DispRefFrame=NED  Temperature=25  MagneticFieldNED=[ 27.5550, -2.4169, -16.0849 ]  MagneticFieldENU=[ -2.4169, 27.5550, 16.0849 ]  SeedDouble=50  SimulateUsing=Code generation  AccelParamsMeasurementRange=4*9.81  AccelParamsResolution=1/(8192*9.81)  AccelParamsConstantBias=[0 0 0]  AccelParamsAxesMisalignment=[0 0 0]  AccelParamsNoiseDensity=1377e-6*[0 0 0]  AccelParamsBiasInstability=[0 0 0]  AccelParamsRandomWalk=[0 0 0]  AccelParamsTemperatureBias=[0 0 0]  AccelParamsTemperatureScaleFactor=[0 0 0]  GyroParamsMeasurementRange=17.4532  GyroParamsResolution=1/3752  GyroParamsConstantBias=[0 0 0]  GyroParamsAxesMisalignment=0  GyroParamsAccelerationBias=[0 0 0]  GyroParamsNoiseDensity=[0 0 0].*0.000  GyroParamsBiasInstability=[0 0 0]  GyroParamsRandomWalk=[0 0 0]  GyroParamsTemperatureBias=[0 0 0]  GyroParamsTemperatureScaleFactor=[0 0 0]  MagParamsMeasurementRange=1600  MagParamsResolution=0.3  MagParamsConstantBias=0  MagParamsAxesMisalignment=[0 0 0]  MagParamsNoiseDensity=[0 0 0]  MagParamsBiasInstability=[0 0 0]  MagParamsRandomWalk=[0 0 0]  MagParamsTemperatureBias=[0 0 0]  MagParamsTemperatureScaleFactor=[0 0 0]
      settings: SourceProductName=Sensor Fusion and Tracking Toolbox
  Integrate Angular Velocity : MATLAB Function  TreatAsAtomicUnit=on  mask{rate=1/1000}
      mask prompts: rate "Sample Rate"
  Manual Switch : ManualSwitch
  Terminator2 : Terminator
  Terminator3 : Terminator
  Transpose3 : Math  Operator=transpose  SaturateOnIntegerOverflow=on
  Transpose4 : Math  Operator=transpose  SaturateOnIntegerOverflow=on
  Transpose5 : Math  Operator=transpose  SaturateOnIntegerOverflow=on
  gyro : Outport
  wires:
  acc/1 -> Transpose4/1
  AHRS/1 -> Terminator2/1
  Add/1 -> Terminator3/1  "error"
  Transpose4/1 -> IMU1/1
  AHRS/2 -> Transpose5/1
  rate/1 -> Manual Switch/2, Add/2, Transpose3/1  "angular rate"
  Integrate Angular Velocity/1(q) -> IMU1/3
  IMU1/3 -> AHRS/3
  Transpose5/1 -> Manual Switch/1, Add/1  "gyro"
  IMU1/1 -> AHRS/1
  Transpose3/1 -> Integrate Angular Velocity/1(av), IMU1/2
  IMU1/2 -> AHRS/2
  Manual Switch/1 -> gyro/1

== system px4_6dof_quadrotor/Attitude Controller/Norm3 ==
  In1 : Inport
  Dot Product : DotProduct  InputSameDT=on  OutDataTypeStr=Inherit: Inherit via internal rule
  Math Function1 : Math  Operator=sqrt  SignedPower=on  SaturateOnIntegerOverflow=on
  Out1 : Outport  VectorParamsAs1DForOutWhenUnconnected=off
  wires:
  Dot Product/1 -> Math Function1/1
  Math Function1/1 -> Out1/1
  In1/1 -> Dot Product/1, Dot Product/2

== system px4_6dof_quadrotor/Attitude Controller/mavros attitude controller ==
  acc_cmd : Inport
  yaw : Inport  Port=2
  MATLAB Function : MATLAB Function  TreatAsAtomicUnit=on
  quat : Outport
  wires:
  MATLAB Function/1(quat) -> quat/1
  acc_cmd/1 -> MATLAB Function/1(vector_acc)
  yaw/1 -> MATLAB Function/2(yaw)

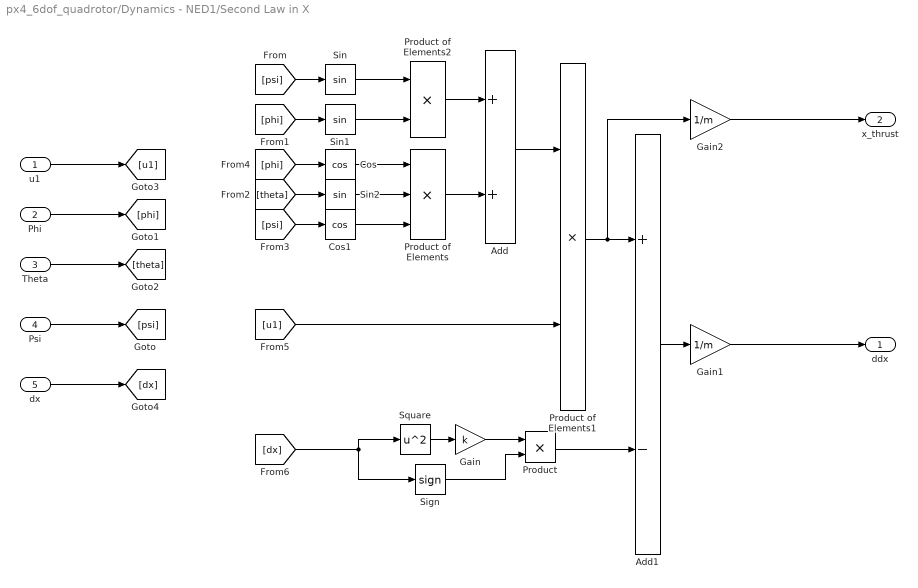
== system px4_6dof_quadrotor/Dynamics - NED1/Second Law in X ==
  u1 : Inport
  Phi : Inport  Port=2
  Theta : Inport  Port=3
  Psi : Inport  Port=4
  dx : Inport  Port=5
  Add : Sum
  Add1 : Sum  Inputs=+-
  Cos : Trigonometry  Operator=cos
  Cos1 : Trigonometry  Operator=cos
  Gain : Gain  Gain=k
  Gain1 : Gain  Gain=1/m
  Gain2 : Gain  Gain=1/m
  Product : Product
  Product of Elements : Product  Inputs=3
  Product of Elements1 : Product
  Product of Elements2 : Product
  Sign : Signum
  Sin : Trigonometry
  Sin1 : Trigonometry
  Sin2 : Trigonometry
  Square : Math  Operator=square  SaturateOnIntegerOverflow=on
  ddx : Outport
  x_thrust : Outport  Port=2
  wires:
  Cos/1 -> Product of Elements/1
  [phi] -> Cos/1
  [psi] -> Cos1/1
  Cos1/1 -> Product of Elements/3
  Sin1/1 -> Product of Elements2/2
  [u1] -> Product of Elements1/2
  Product of Elements/1 -> Add/2
  Product of Elements1/1 -> Gain2/1, Add1/1
  Add/1 -> Product of Elements1/1
  [theta] -> Sin2/1
  Sin2/1 -> Product of Elements/2
  Product of Elements2/1 -> Add/1
  [psi] -> Sin/1
  Sin/1 -> Product of Elements2/1
  [phi] -> Sin1/1
  Add1/1 -> Gain1/1
  Psi/1 -> [psi]
  Phi/1 -> [phi]
  Theta/1 -> [theta]
  u1/1 -> [u1]
  dx/1 -> [dx]
  Gain1/1 -> ddx/1
  Square/1 -> Gain/1
  [dx] -> Square/1, Sign/1
  Gain/1 -> Product/1
  Sign/1 -> Product/2
  Product/1 -> Add1/2
  Gain2/1 -> x_thrust/1

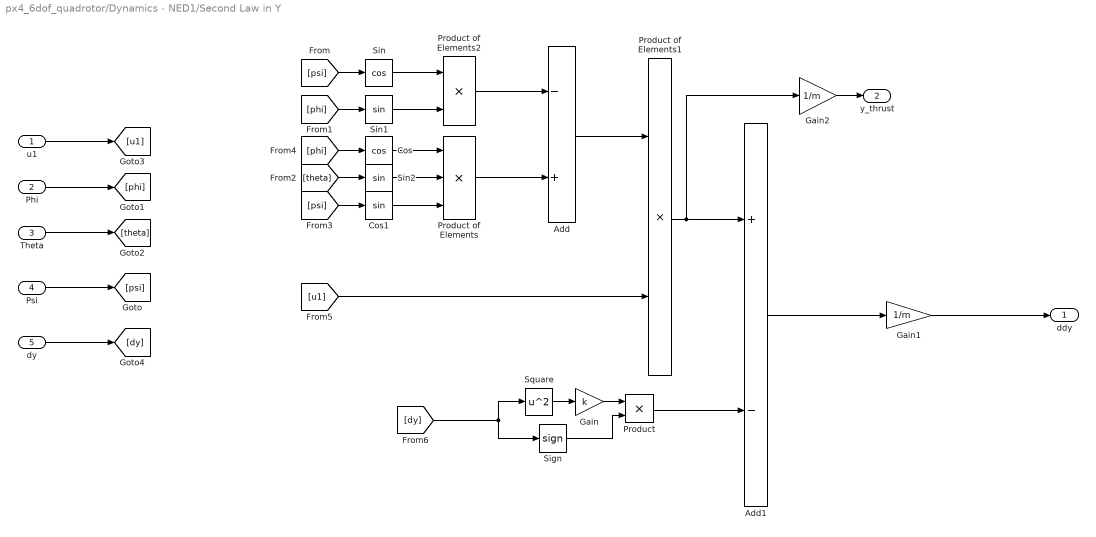
== system px4_6dof_quadrotor/Dynamics - NED1/Second Law in Y ==
  u1 : Inport
  Phi : Inport  Port=2
  Theta : Inport  Port=3
  Psi : Inport  Port=4
  dy : Inport  Port=5
  Add : Sum  Inputs=-+
  Add1 : Sum  Inputs=+-
  Cos : Trigonometry  Operator=cos
  Cos1 : Trigonometry
  Gain : Gain  Gain=k
  Gain1 : Gain  Gain=1/m
  Gain2 : Gain  Gain=1/m
  Product : Product
  Product of Elements : Product  Inputs=3
  Product of Elements1 : Product
  Product of Elements2 : Product
  Sign : Signum
  Sin : Trigonometry  Operator=cos
  Sin1 : Trigonometry
  Sin2 : Trigonometry
  Square : Math  Operator=square  SaturateOnIntegerOverflow=on
  ddy : Outport
  y_thrust : Outport  Port=2
  wires:
  dy/1 -> [dy]
  u1/1 -> [u1]
  Theta/1 -> [theta]
  Phi/1 -> [phi]
  Psi/1 -> [psi]
  Add1/1 -> Gain1/1
  [phi] -> Sin1/1
  Sin/1 -> Product of Elements2/1
  [psi] -> Sin/1
  Product of Elements2/1 -> Add/1
  Sin2/1 -> Product of Elements/2
  [theta] -> Sin2/1
  Add/1 -> Product of Elements1/1
  Product of Elements1/1 -> Gain2/1, Add1/1
  Product of Elements/1 -> Add/2
  [u1] -> Product of Elements1/2
  Sin1/1 -> Product of Elements2/2
  Cos1/1 -> Product of Elements/3
  [psi] -> Cos1/1
  [phi] -> Cos/1
  Cos/1 -> Product of Elements/1
  Gain1/1 -> ddy/1
  [dy] -> Square/1, Sign/1
  Square/1 -> Gain/1
  Sign/1 -> Product/2
  Gain/1 -> Product/1
  Product/1 -> Add1/2
  Gain2/1 -> y_thrust/1

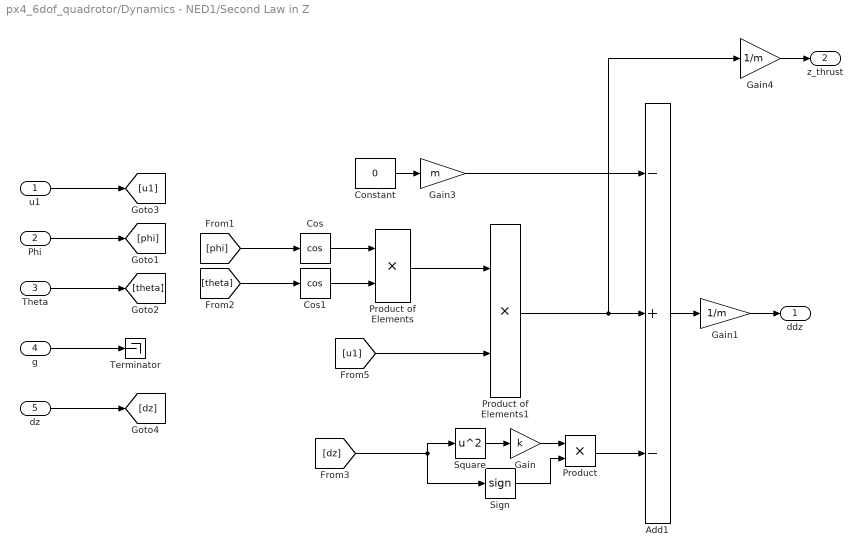
== system px4_6dof_quadrotor/Dynamics - NED1/Second Law in Z ==
  u1 : Inport
  Phi : Inport  Port=2
  Theta : Inport  Port=3
  g : Inport  Port=4
  dz : Inport  Port=5
  Add1 : Sum  Inputs=-+-
  Constant : Constant  Value=0
  Cos : Trigonometry  Operator=cos
  Cos1 : Trigonometry  Operator=cos
  Gain : Gain  Gain=k
  Gain1 : Gain  Gain=1/m
  Gain3 : Gain  Gain=m
  Gain4 : Gain  Gain=1/m
  Product : Product
  Product of Elements : Product
  Product of Elements1 : Product
  Sign : Signum
  Square : Math  Operator=square  SaturateOnIntegerOverflow=on
  Terminator : Terminator
  ddz : Outport
  z_thrust : Outport  Port=2
  wires:
  Product of Elements1/1 -> Gain4/1, Add1/2
  [u1] -> Product of Elements1/2
  Add1/1 -> Gain1/1
  g/1 -> Terminator/1
  Phi/1 -> [phi]
  Theta/1 -> [theta]
  u1/1 -> [u1]
  dz/1 -> [dz]
  Product of Elements/1 -> Product of Elements1/1
  Cos/1 -> Product of Elements/1
  [phi] -> Cos/1
  Cos1/1 -> Product of Elements/2
  [theta] -> Cos1/1
  Gain1/1 -> ddz/1
  [dz] -> Sign/1, Square/1
  Square/1 -> Gain/1
  Sign/1 -> Product/2
  Gain/1 -> Product/1
  Product/1 -> Add1/3
  Gain4/1 -> z_thrust/1
  Constant/1 -> Gain3/1
  Gain3/1 -> Add1/1

== matlab function px4_6dof_quadrotor/Attitude Controller/mavros attitude controller/MATLAB Function ==
  data: vector_acc input; quat output size=[1 4]; yaw input
function quat = fcn(vector_acc,yaw)

proj_xb_des = [cos(yaw) sin(yaw) 0];

zb_des = vector_acc / norm(vector_acc) ;
yb_des = cross(zb_des,proj_xb_des) / norm(cross(zb_des,proj_xb_des));
xb_des = cross(yb_des,zb_des) / norm(cross(yb_des,zb_des));

rotmat = [xb_des(1) yb_des(1) zb_des(1);xb_des(2) yb_des(2) zb_des(2);xb_des(3) yb_des(3) zb_des(3)];

quat = rotm2quat(rotmat);

== matlab function px4_6dof_quadrotor/Mixer/MATLAB Function ==
  data: mat input; y output; vect input
function y = fcn(mat,vect)
y = mat\vect;

== matlab function px4_6dof_quadrotor/Subsystem/Integrate Angular Velocity ==
  data: av input; q output; rate parameter
function q = integrateAngVel(av, rate)
%INTEGRATEANGVEL Integrate angular velocity to a quaternion
%  Treat Angular Velocity as an incremental rotation vector.

%   Copyright 2019 The MathWorks, Inc.   

persistent orient
if isempty(orient)
    % Initial orientation is the identity quaternion.
    orient = cast(quaternion(1,0,0,0), 'like', av);
end

% Convert angular velocity to a rotation vector.
rv = quaternion(av*(1/rate), 'rotvec');
orient = rv * orient;
q = compact(orient);
